simulink model "prototype1"  (R2016b)
settings: Solver=VariableStepAuto  StartTime=0.0  StopTime=10.0  RelTol=1e-3
libraries: simulink x1
settings Model: Creator=jadevarelle  LastModifiedBy=jadevarelle

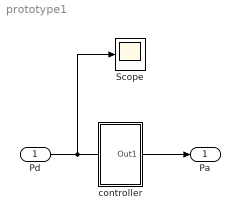
== system prototype1 ==
  Pd : Inport
  Scope : Scope
  "controller " : Subsystem
  Pa : Outport
  wires:
  Pd/1 -> Scope/1
  "controller "/1(Out1) -> Pa/1

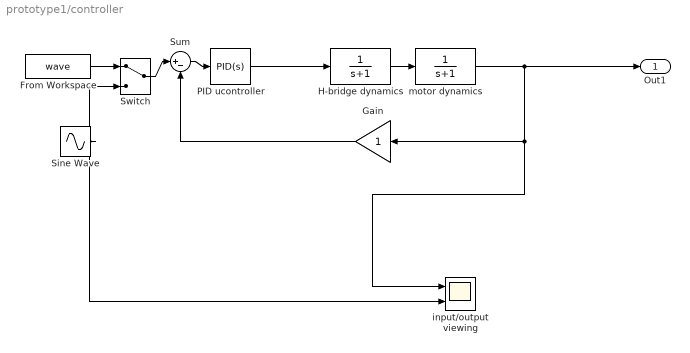
== system prototype1/controller  ==
  From Workspace : FromWorkspace  VariableName=wave  SampleTime=0
  Gain : Gain
  H-bridge dynamics : TransferFcn  Denominator=[1 1]
  PID ucontroller : simulink/Continuous/PID Controller  Controller=PID  TimeDomain=Continuous-time  SampleTime=-1  IntegratorMethod=Forward Euler  FilterMethod=Forward Euler  Form=Parallel  UseFilter=on  ControllerParametersSource=internal  P=1  I=0  D=0  N=100  InitialConditionSource=internal  InitialConditionForIntegrator=0  InitialConditionForFilter=0  ExternalReset=none  LimitOutput=off  UpperSaturationLimit=inf  LowerSaturationLimit=-inf  LinearizeAsGain=on  AntiWindupMode=none  Kb=1  TrackingMode=off  Kt=1  PParamMin=[]  PParamMax=[]  IParamMin=[]  IParamMax=[]  DParamMin=[]  DParamMax=[]  NParamMin=[]  NParamMax=[]  KbParamMin=[]  KbParamMax=[]  KtParamMin=[]  KtParamMax=[]  POutMin=[]  POutMax=[]  IOutMin=[]  IOutMax=[]  DOutMin=[]  DOutMax=[]  NOutMin=[]  NOutMax=[]  KbOutMin=[]  KbOutMax=[]  KtOutMin=[]  KtOutMax=[]  IntegratorOutMin=[]  IntegratorOutMax=[]  FilterOutMin=[]  FilterOutMax=[]  SumOutMin=[]  SumOutMax=[]  SumI1OutMin=[]  SumI1OutMax=[]  SumI2OutMin=[]  SumI2OutMax=[]  SumI3OutMin=[]  SumI3OutMax=[]  SumDOutMin=[]  SumDOutMax=[]  SaturationOutMin=[]  SaturationOutMax=[]  IntegratorContinuousStateAttributes=''  IntegratorStateMustResolveToSignalObject=off  IntegratorRTWStateStorageClass=Auto  FilterContinuousStateAttributes=''  FilterStateMustResolveToSignalObject=off  FilterRTWStateStorageClass=Auto  DifferentiatorICPrevScaledInput=0  DifferentiatorOutMin=[]  DifferentiatorOutMax=[]
  Sine Wave : Sin  SampleTime=0
  Sum : Sum  Inputs=|+-
  Switch : ManualSwitch
  "input/output viewing " : Scope  NumInputPorts=2
  motor dynamics : TransferFcn  Denominator=[1 1]
  Out1 : Outport
  wires:
  Sine Wave/1 -> "input/output viewing "/2, Switch/2
  motor dynamics/1 -> Gain/1, "input/output viewing "/1, Out1/1
  Sum/1 -> PID ucontroller/1
  Switch/1 -> Sum/1
  H-bridge dynamics/1 -> motor dynamics/1
  PID ucontroller/1 -> H-bridge dynamics/1
  Gain/1 -> Sum/2
  From Workspace/1 -> Switch/1
